simulink model "Narnia_model"  (R2023b)
settings: Solver=VariableStepAuto  StartTime=0.0  StopTime=inf  FixedStep=1  RelTol=1e-3  EnableMultiTasking=on
values from neighbouring files (symbols this model uses):
  P = 0.2    [train_agent.m]
  Tf = 24    [train_agent.m]
undefined symbols (not defined in the file or in its folder): A, B, C, DiscIntNeverNeededParam, E, HeatLimit
libraries: simulink x4, eeGeneralControl x1, rllib x1
settings Model: Creator=The MathWorks, Inc.  LastModifiedBy=hdt
settings SolverCC: AlgebraicLoopSolver=TrustRegion  MinimalZcImpactIntegration=on
settings DataIOCC: LimitDataPoints=on  SaveFormat=Array
settings OptimizationCC: ReuseModelBlockBuffer=off  LifeSpan=inf
settings DebuggingCC: UnconnectedInputMsg=warning  UnconnectedOutputMsg=warning  UnconnectedLineMsg=warning  SFUnexpectedBacktrackingDiag=warning  SFNoUnconditionalDefaultTransitionDiag=warning  SFExecutionAtInitializationDiag=none  ArithmeticOperatorsInVariantConditions=warning
settings HardwareCC: ProdBitPerPointer=32  ProdBitPerSizeT=32  ProdBitPerPtrDiffT=32  ProdLargestAtomicFloat=None  ProdIntDivRoundTo=Undefined  ProdEndianess=Unspecified  ProdWordSize=32  ProdHWDeviceType=32-bit Generic
settings ModelReferenceCC: EnableRefExpFcnMdlSchedulingChecks=on  PropagateSignalLabelsOutOfModel=off
settings SFSimCC: SimUseLocalCustomCode=off  CustomCodeUndefinedFunction=UseInterfaceOnly
settings RTWCC: RTWUseLocalCustomCode=off
settings CodeAppCC: StateflowObjectComments=on
settings GRTTargetCC: TargetLangStandard=C89/C90 (ANSI)
settings ConfigComp: CovMetricSettings=dw  CovSaveCumulativeToWorkspaceVar=on  CovSaveSingleToWorkspaceVar=on  CovExternalEMLEnable=off  CovSFcnEnable=off

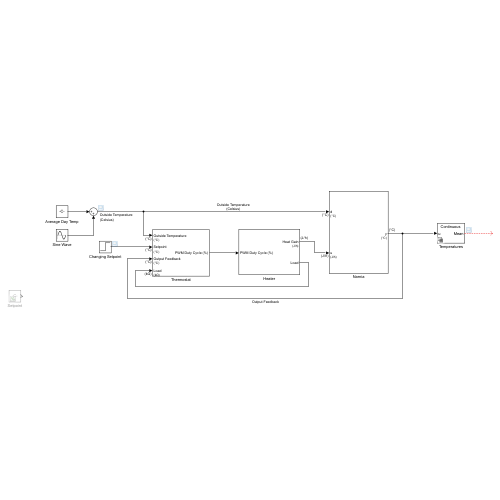
[thumbnail: Simulink's stored preview of the top-level diagram]
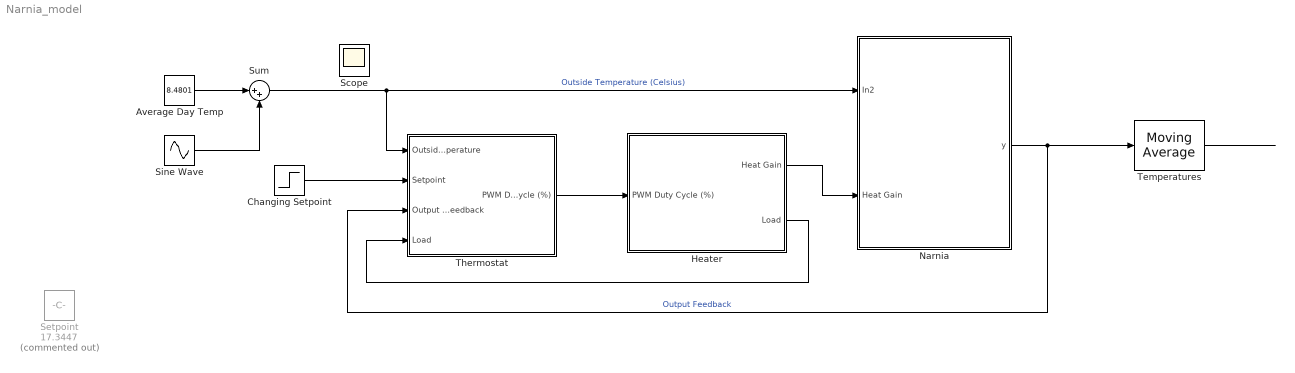
== system Narnia_model ==
  Average Day Temp : Constant  Value=8.4801
  Changing Setpoint : Step  Time=Tf/2  Before=16.4102  After=17.7136  SampleTime=0  VectorParams1D=off
  Heater : Subsystem
  Narnia : Subsystem
  Setpoint : Constant  Commented=on  Value=17.3447
  Sine Wave : Sin  Amplitude=4  Frequency=pi/12  SampleTime=0
  Sum : Sum  Inputs=|++
  Temperatures : eeGeneralControl/Moving Average  VariantControl=Variant1  LabelModeActiveChoice=Continuous  f=2  x0=0  BufferSize=8192  Ts=0
      settings: LibrarySourceBlock=ee_sl_lib/General Control/Moving Average
  Thermostat : Subsystem
  Scope : Scope
  wires:
  Thermostat/1(PWM Duty Cycle (%)) -> Heater/1(PWM Duty Cycle (%))
  Heater/1(Heat Gain) -> Narnia/2(Heat Gain)
  Narnia/1(y) -> Temperatures/1, Thermostat/3(Output Feedback)  "Output Feedback"
  Changing Setpoint/1 -> Thermostat/2(Setpoint)
  Sine Wave/1 -> Sum/2
  Average Day Temp/1 -> Sum/1
  Sum/1 -> Thermostat/1(Outside Temperature), Narnia/1(In2)  "Outside Temperature (Celsius)"
  Temperatures/1 -> ?
  Heater/2(Load) -> Thermostat/4(Load)

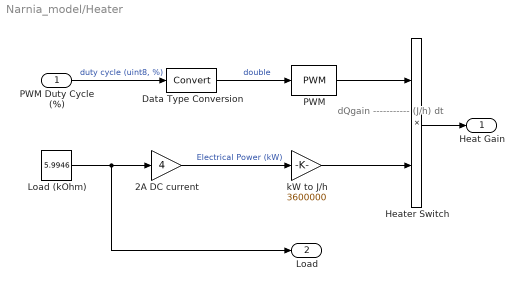
== system Narnia_model/Heater ==
  note: dQgain
      | ----------- (J/h)
      |    dt
  PWM Duty Cycle (%) : Inport
  2A DC current : Gain  Gain=4
  Data Type Conversion : DataTypeConversion  SaturateOnIntegerOverflow=off  RndMeth=Floor
  Heater Switch : Product  RndMeth=Zero
  Load (kOhm) : Constant  Value=5.9946
  PWM : simulink/Discontinuities/PWM  DisableCoverage=on  Period=P  InitialDelay=0  DisallowZeroDutyCycle=off  RunAtFixedTimeIntervals=off  SampleTime=0.1
  kW to J/h : Gain  Gain=3600000
  Heat Gain : Outport  Unit=joule/hour  VectorParamsAs1DForOutWhenUnconnected=off
  Load : Outport  Port=2
  wires:
  PWM/1 -> Heater Switch/1
  Heater Switch/1 -> Heat Gain/1
  Load (kOhm)/1 -> Load/1, 2A DC current/1
  kW to J/h/1 -> Heater Switch/2
  Data Type Conversion/1 -> PWM/1  "double"
  PWM Duty Cycle (%)/1 -> Data Type Conversion/1  "duty cycle (uint8, %)"
  2A DC current/1 -> kW to J/h/1  "Electrical Power (kW)"

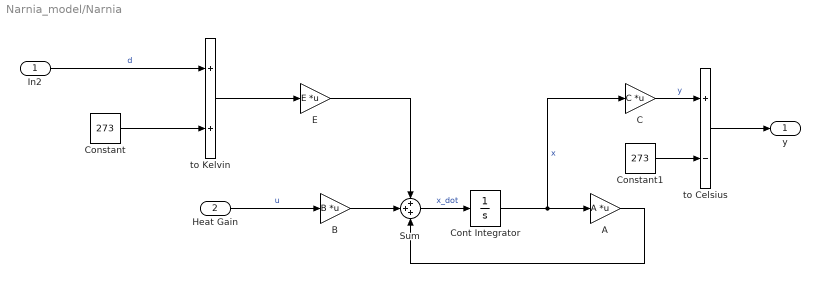
== system Narnia_model/Narnia ==
  In2 : Inport  Unit=Celsius
  Heat Gain : Inport  Port=2  Unit=J/h
  A : Gain  Gain=A  Multiplication=Matrix(K*u)
  B : Gain  Gain=B  Multiplication=Matrix(K*u)
  C : Gain  Gain=C  Multiplication=Matrix(K*u)
  Constant : Constant  Value=273
  Constant1 : Constant  Value=273
  Cont Integrator : Integrator  InitialCondition=289.3746
  E : Gain  Gain=E  Multiplication=Matrix(K*u)
  Sum : Sum  Inputs=+++
  to Celsius : Sum  Inputs=+-
  to Kelvin : Sum
  y : Outport  Unit=°C
  wires:
  Heat Gain/1 -> B/1  "u"
  B/1 -> Sum/2
  A/1 -> Sum/3
  Sum/1 -> Cont Integrator/1  "x_dot"
  Cont Integrator/1 -> C/1, A/1  "x"
  E/1 -> Sum/1
  In2/1 -> to Kelvin/1  "d"
  C/1 -> to Celsius/1  "y"
  Constant/1 -> to Kelvin/2
  to Kelvin/1 -> E/1
  to Celsius/1 -> y/1
  Constant1/1 -> to Celsius/2

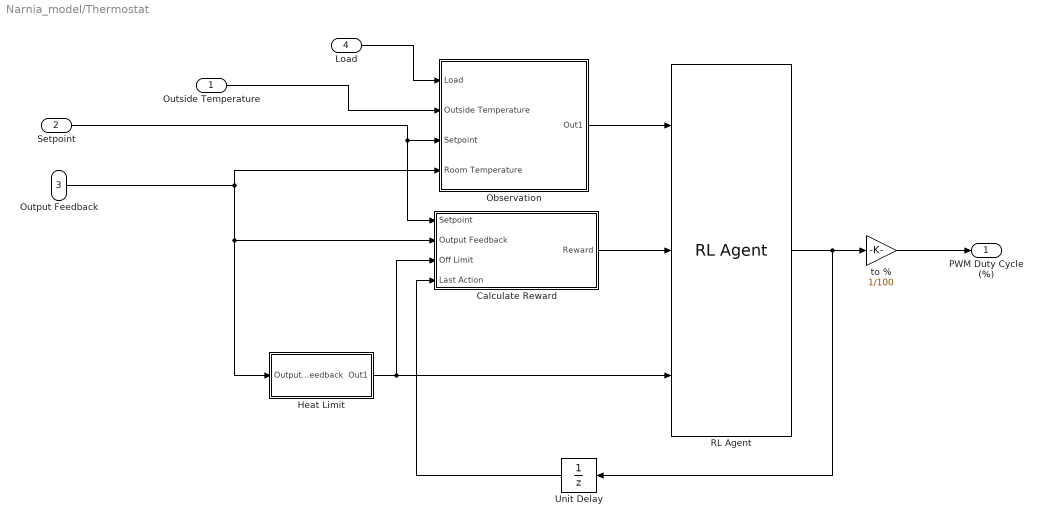
== system Narnia_model/Thermostat ==
  Outside Temperature : Inport  Unit=°C
  Setpoint : Inport  Port=2  Unit=°C
  Output Feedback : Inport  Port=3  Unit=°C
  Load : Inport  Port=4  Unit=kΩ
  Calculate Reward : Subsystem
  Heat Limit : Subsystem
  Observation : Subsystem
  RL Agent : rllib/RL Agent  Agent=default_agent  ExternalActionAsInput=off  ProvideLastAction=off  ProvideCumRwd=off  TreatAsDirectFeedthrough=on  UseStrictObservationDataTypes=off
  Unit Delay : UnitDelay  SampleTime=-1  HasFrameUpgradeWarning=on
  to % : Gain  Gain=1/100
  PWM Duty Cycle (%) : Outport  VectorParamsAs1DForOutWhenUnconnected=off
  wires:
  Setpoint/1 -> Calculate Reward/1(Setpoint), Observation/3(Setpoint)
  Output Feedback/1 -> Observation/4("    Room Temperature"), Heat Limit/1(Output Feedback), Calculate Reward/2(Output Feedback)
  Outside Temperature/1 -> Observation/2(Outside Temperature)
  Observation/1(Out1) -> RL Agent/1
  Calculate Reward/1(Reward) -> RL Agent/2
  Heat Limit/1(Out1) -> Calculate Reward/3(Off Limit), RL Agent/3
  RL Agent/1 -> Unit Delay/1, to %/1
  to %/1 -> PWM Duty Cycle (%)/1
  Unit Delay/1 -> Calculate Reward/4(Last Action)
  Load/1 -> Observation/1(Load)

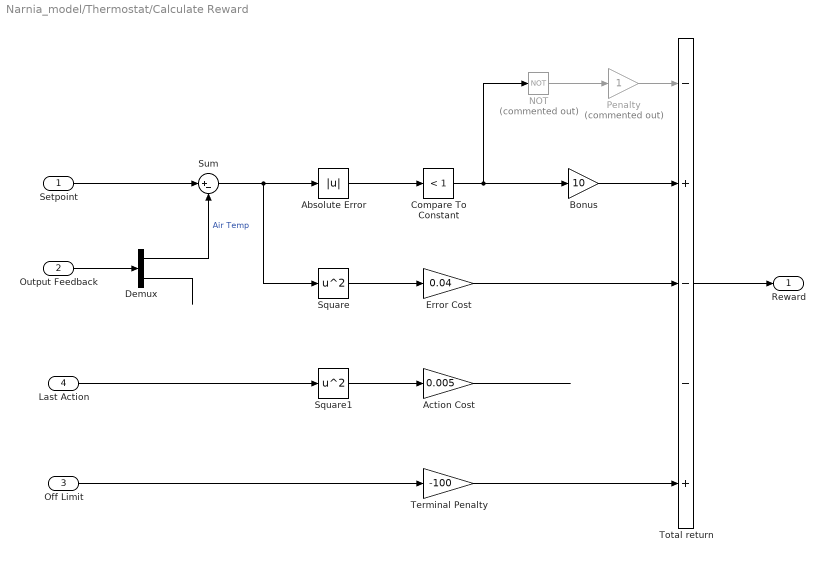
== system Narnia_model/Thermostat/Calculate Reward ==
  Setpoint : Inport
  Output Feedback : Inport  Port=2
  Off Limit : Inport  Port=3
  Last Action : Inport  Port=4
  Absolute Error : Abs  SaturateOnIntegerOverflow=off
  Action Cost : Gain  Gain=0.005
  Bonus : Gain  Gain=10
  Compare To Constant : simulink/Logic and Bit Operations/Compare To Constant  relop=<  const=1  OutDataTypeStr=boolean
  Demux : Demux  Outputs=2
  Error Cost : Gain  Gain=0.04
  NOT : Logic  Commented=on  Operator=NOT  IconShape=distinctive  AllPortsSameDT=off  OutDataTypeStr=boolean
  Penalty : Gain  Commented=on
  Square : Math  Operator=square
  Square1 : Math  Operator=square
  Sum : Sum  Inputs=|+-
  Terminal Penalty : Gain  Gain=-100
  Total return : Sum  Inputs=-+--+
  Reward : Outport
  wires:
  Setpoint/1 -> Sum/1
  Total return/1 -> Reward/1
  Terminal Penalty/1 -> Total return/5
  Off Limit/1 -> Terminal Penalty/1
  Sum/1 -> Square/1, Absolute Error/1
  Output Feedback/1 -> Demux/1
  Absolute Error/1 -> Compare To Constant/1
  Bonus/1 -> Total return/2
  Compare To Constant/1 -> NOT/1, Bonus/1
  Penalty/1 -> Total return/1
  NOT/1 -> Penalty/1
  Demux/1 -> Sum/2  "Air Temp"
  Demux/2 -> ?
  Error Cost/1 -> Total return/3
  Square/1 -> Error Cost/1
  Square1/1 -> Action Cost/1
  Action Cost/1 -> ?
  Last Action/1 -> Square1/1

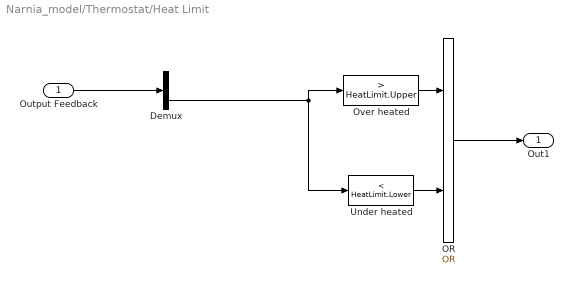
== system Narnia_model/Thermostat/Heat Limit ==
  Output Feedback : Inport
  Demux : Demux  Outputs=2
  OR : Logic  Operator=OR  IconShape=distinctive  AllPortsSameDT=off  OutDataTypeStr=boolean
  Over heated : simulink/Logic and Bit Operations/Compare To Constant  relop=>  const=HeatLimit.Upper  OutDataTypeStr=boolean
  Under heated : simulink/Logic and Bit Operations/Compare To Constant  relop=<  const=HeatLimit.Lower  OutDataTypeStr=boolean
  Out1 : Outport
  wires:
  Demux/2 -> Under heated/1, Over heated/1
  Under heated/1 -> OR/2
  Over heated/1 -> OR/1
  OR/1 -> Out1/1
  Output Feedback/1 -> Demux/1

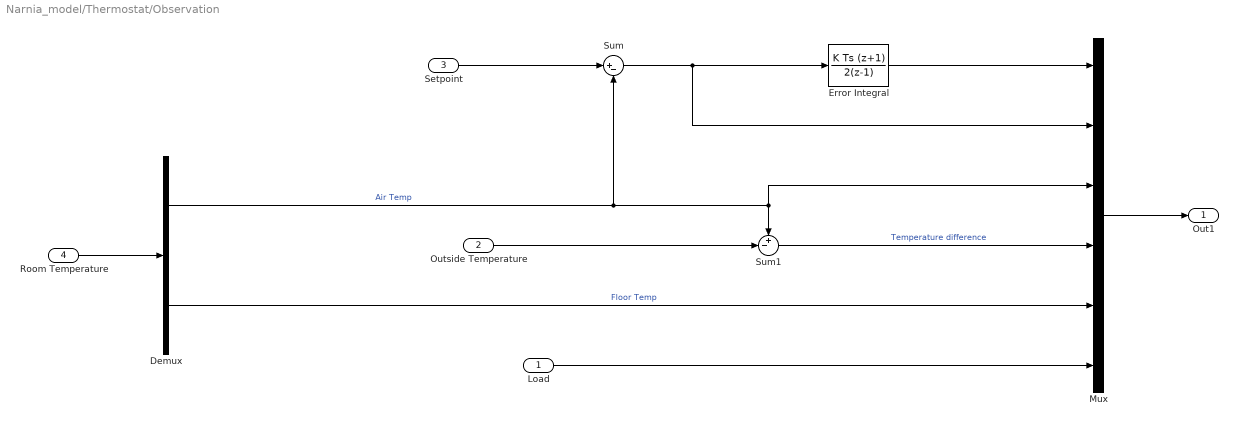
== system Narnia_model/Thermostat/Observation ==
  Load : Inport
  Outside Temperature : Inport  Port=2
  Setpoint : Inport  Port=3
  "    Room Temperature" : Inport  Port=4
  Demux : Demux  Outputs=2
  Error Integral : DiscreteIntegrator  IntegratorMethod=Integration: Trapezoidal  SampleTime=-1  ICPrevOutput=DiscIntNeverNeededParam  ICPrevScaledInput=DiscIntNeverNeededParam
  Mux : Mux  Inputs=6
  Sum : Sum  Inputs=|+-
  Sum1 : Sum  Inputs=+-|
  Out1 : Outport
  wires:
  Outside Temperature/1 -> Sum1/2
  Setpoint/1 -> Sum/1
  Demux/1 -> Sum/2, Sum1/1, Mux/3  "Air Temp"
  Error Integral/1 -> Mux/1
  Mux/1 -> Out1/1
  Sum/1 -> Error Integral/1, Mux/2
  Sum1/1 -> Mux/4  "Temperature difference"
  "    Room Temperature"/1 -> Demux/1
  Demux/2 -> Mux/5  "Floor Temp"
  Load/1 -> Mux/6
